simulink model "vipmosaicking"  (R2015b)
settings: Solver=FixedStepDiscrete  StartTime=0.0  StopTime=inf  RelTol=1e-3
undefined symbols (not defined in the file or in its folder): fspecial, gray, imresize, Rec, SDTV
libraries: simulink x5, visiongeotforms x4, visionsinks x2, visiontextngfix x2, visionanalysis x1, visionstatistics x1, vipmisc x1, visionconversions x1, visionsources x1, dspvision x1
settings Model: FPTRunName=Active  Creator=The MathWorks, Inc.  LastModifiedBy=The MathWorks, Inc.
settings DataIOCC: SaveFormat=Array  SaveOutput=off  SignalLogging=off  SaveTime=off
settings OptimizationCC: ExpressionDepthLimit=2147483647  InitFltsAndDblsToZero=on  EfficientMapNaN2IntZero=off
settings DebuggingCC: CheckSSInitialOutputMsg=off  UnderspecifiedInitializationDetection=Classic  MergeDetectMultiDrivingBlocksExec=none  SolverPrmCheckMsg=warning  InheritedTsInSrcMsg=none  ParameterPrecisionLossMsg=none  FcnCallInpInsideContextMsg=UseLocalSettings  StateNameClashWarn=warning
settings HardwareCC: ProdBitPerPointer=32  ProdLargestAtomicFloat=None  ProdIntDivRoundTo=Undefined  ProdEndianess=Unspecified  ProdWordSize=32  ProdHWDeviceType=32-bit Generic  TargetBitPerLong=64  TargetBitPerPointer=64  TargetLongLongMode=on  TargetIntDivRoundTo=Zero  TargetEndianess=LittleEndian  TargetWordSize=64  TargetHWDeviceType=Generic->MATLAB Host Computer  ProdEqTarget=off
settings GRTTargetCC: GeneratePreprocessorConditionals=Disable all  CombineOutputUpdateFcns=off  GRTInterface=on
settings ConfigComp: CovModelRefEnable=Off  CovSFcnEnable=off

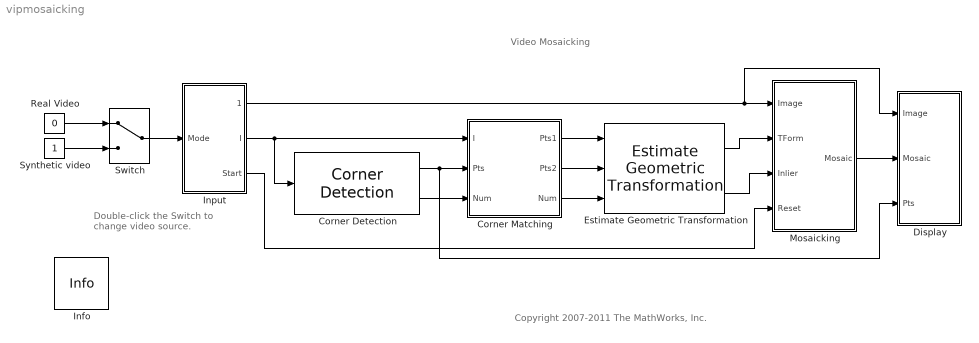
== system vipmosaicking ==
  note: Video Mosaicking
  note: Double-click the Switch to
      | change video source.
  note: Copyright 2007-2011 The MathWorks, Inc.
  Corner Detection : visionanalysis/Corner Detection  method=Local intensity comparison (Rosen & Drummond)  factor=0.04  filter=fspecial('gaussian', [1 5], 1.5)  thrInten=0.1  thrAngle=157.5  output=Obsolete9b  outputInUse=Corner location  maxNum=75  thrMetric=0.001  neighborSize=[21 21]  isOutVarDim=off  accumMode=Binary point scaling  accumWordLength=32  accumFracLength=0  prodOutputMode=Binary point scaling  prodOutputWordLength=32  prodOutputFracLength=0  memoryMode=Binary point scaling  memoryWordLength=32  memoryFracLength=0  firstCoeffMode=Specify word length  firstCoeffWordLength=16  firstCoeffFracLength=16  roundingMode=Floor  overflowMode=off
  Corner Matching : Subsystem  mask(Corner Matching){winLen=9, maxNum=75, threshold=81}
      mask prompts: winLen "Block size used in corner matching:"; maxNum "Maximum number of points:"; threshold "Maximum feature difference for matching points:"
      mask help: Find out matching corners in the current and previous video frames.
  Display : Subsystem
  Estimate Geometric Transformation : visiongeotforms/Estimate Geometric Transformation  tformType=Nonreflective similarity  isRandomSampling=on  algMethod=Random Sample Consensus (RANSAC)  numMethod=Specified value  isStopSampling=off  percentStop=75  distanceAlg=1  distanceGeo=2.5  sampleNum=1000  maxSampleNum=2000  desiredConfidence=99.9  isRefineTForm=off  isOutputInlier=on  outDT4IntInput=Obsolete10a  outDT4IntInputActive=Single  isVarSizeAllowed=off  isReleaseMode=on
  Info : vipmisc/Info  SystemSampleTime=-1
  Input : Subsystem
  Mosaicking : Subsystem  mask(Mosaicking){sizePano=[400 670], originPano=[5 60]}
      mask prompts: sizePano "Size of the mosaic image:"; originPano "Initial image placement (top-left image boundary):"
      mask help: Overlay video frames to create mosaic image.
  Real Video : Constant  Value=0
  Switch : ManualSwitch
  Synthetic video : Constant
  wires:
  Input/1(Image) -> Display/1(Image), Mosaicking/1(Image)
  Input/3(Start) -> Mosaicking/4(Reset)
  Corner Detection/1 -> Display/3(Pts), Corner Matching/2(Pts)
  Corner Detection/2 -> Corner Matching/3(Num)
  Input/2(I) -> Corner Matching/1(I), Corner Detection/1
  Mosaicking/1(Mosaic) -> Display/2(Mosaic)
  Corner Matching/1(Pts1) -> Estimate Geometric Transformation/1
  Corner Matching/2(Pts2) -> Estimate Geometric Transformation/2
  Corner Matching/3("Num ") -> Estimate Geometric Transformation/3
  Estimate Geometric Transformation/2 -> Mosaicking/3(Inlier)
  Estimate Geometric Transformation/1 -> Mosaicking/2(TForm)
  Real Video/1 -> Switch/1
  Synthetic video/1 -> Switch/2
  Switch/1 -> Input/1(Mode)

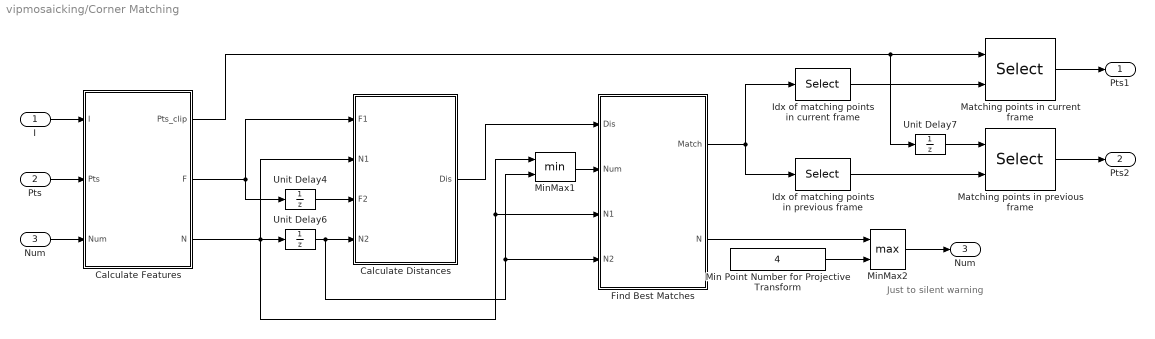
== system vipmosaicking/Corner Matching ==
  note: Just to
      | silent warning
  I : Inport
  Pts : Inport  Port=2
  Num : Inport  Port=3
  Calculate Distances : Subsystem  TreatAsAtomicUnit=on  mask{maxNum=maxNum}
      mask prompts: maxNum "Maximum data number:"
      settings: AttributesFormatString=between features.
  Calculate Features : Subsystem  TreatAsAtomicUnit=on  mask{winLen=winLen, maxNum=maxNum}
      mask prompts: winLen "Neighborhood size:"; maxNum "Maximum number of features:"
  Find Best Matches : Subsystem  TreatAsAtomicUnit=on  mask{maxNum=maxNum, threshold=threshold}
      mask prompts: maxNum "Maximum data number:"
      settings: AttributesFormatString=between the features\nin the current and previous frames
  Idx of matching points in current frame : Selector  NumberOfDimensions=2  IndexMode=Zero-based  InputPortWidth=2  IndexOptions=Select all,Index vector (dialog)  Indices=0,0  OutputSizes=1,1
  Idx of matching points in previous frame : Selector  NumberOfDimensions=2  IndexMode=Zero-based  InputPortWidth=2  IndexOptions=Select all,Index vector (dialog)  Indices=1,1  OutputSizes=1,1
  Matching points in current frame : Selector  NumberOfDimensions=2  IndexMode=Zero-based  InputPortWidth=2  IndexOptions=Index vector (port),Select all  Indices=0,1  OutputSizes=1,1
  Matching points in previous frame : Selector  NumberOfDimensions=2  IndexMode=Zero-based  InputPortWidth=2  IndexOptions=Index vector (port),Select all  Indices=0,1  OutputSizes=1,1
  Min Point Number for Projective Transform : Constant  Value=4  OutDataTypeStr=Inherit: Inherit via back propagation
  MinMax1 : MinMax  Inputs=2
  MinMax2 : MinMax  Function=max  Inputs=2  OutDataTypeStr=Inherit: Inherit via back propagation
  Unit Delay4 : UnitDelay  SampleTime=-1
  Unit Delay6 : UnitDelay  SampleTime=-1
  Unit Delay7 : UnitDelay  SampleTime=-1
  Pts1 : Outport
  Pts2 : Outport  Port=2
  "Num " : Outport  Port=3
  wires:
  Calculate Features/2(F) -> Calculate Distances/1(F1), Unit Delay4/1
  Calculate Features/3(N) -> Calculate Distances/2(N1), Unit Delay6/1, MinMax1/1, Find Best Matches/3(N1)
  Calculate Features/1(Pts_clip) -> Unit Delay7/1, Matching points in current frame/1
  Num/1 -> Calculate Features/3(Num)
  Unit Delay6/1 -> Calculate Distances/4(N2), MinMax1/2, Find Best Matches/4(N2)
  Unit Delay4/1 -> Calculate Distances/3(F2)
  Matching points in previous frame/1 -> Pts2/1
  Matching points in current frame/1 -> Pts1/1
  Unit Delay7/1 -> Matching points in previous frame/1
  Idx of matching points in current frame/1 -> Matching points in current frame/2
  Idx of matching points in previous frame/1 -> Matching points in previous frame/2
  Find Best Matches/1(Match) -> Idx of matching points in previous frame/1, Idx of matching points in current frame/1
  Calculate Distances/1(Dis) -> Find Best Matches/1(Dis)
  I/1 -> Calculate Features/1(I)
  Pts/1 -> Calculate Features/2(Pts)
  Min Point Number for Projective Transform/1 -> MinMax2/2
  Find Best Matches/2(N) -> MinMax2/1
  MinMax2/1 -> "Num "/1
  MinMax1/1 -> Find Best Matches/2(Num)

== system vipmosaicking/Display ==
  Image : Inport
  Mosaic : Inport  Port=2
  Pts : Inport  Port=3
  Corners : visionsinks/Video Viewer  inputType=Obsolete7b  imagePorts=One multidimensional signal  useColorMap=off  colormapValue=gray(256)  specRange=off  minInputVal=0  maxInputVal=255  FigPos=[34 421 347 276]  AxisZoom=on  trueSizedOnce=on  OpenAtMdlStart=on  DefaultConfigurationName=vipscopes.VideoViewerScopeCfg
  Draw Corners : visiontextngfix/Draw Markers  shape=Circle  size=3  fill=off  fillClrSource=Specify via dialog  display=User-specified value  intensity=155  color=[1 0 0]  opacity=1  viewport=Entire image  antialiasing=off  inType=Obsolete  imagePorts=One multidimensional signal  prodOutputMode=Binary point scaling  prodOutputWordLength=32  prodOutputFracLength=14  memoryMode=Specify word length  memoryWordLength=16  memoryFracLength=15  roundingMode=Floor  overflowMode=off
  "Mosaic " : visionsinks/Video Viewer  inputType=Obsolete7b  imagePorts=One multidimensional signal  useColorMap=off  colormapValue=gray(256)  specRange=off  minInputVal=0  maxInputVal=255  FigPos=[316 541 689 427]  AxisZoom=on  trueSizedOnce=on  OpenAtMdlStart=on  DefaultConfigurationName=vipscopes.VideoViewerScopeCfg
  wires:
  Mosaic/1 -> "Mosaic "/1
  Image/1 -> Draw Corners/1
  Draw Corners/1 -> Corners/1
  Pts/1 -> Draw Corners/2

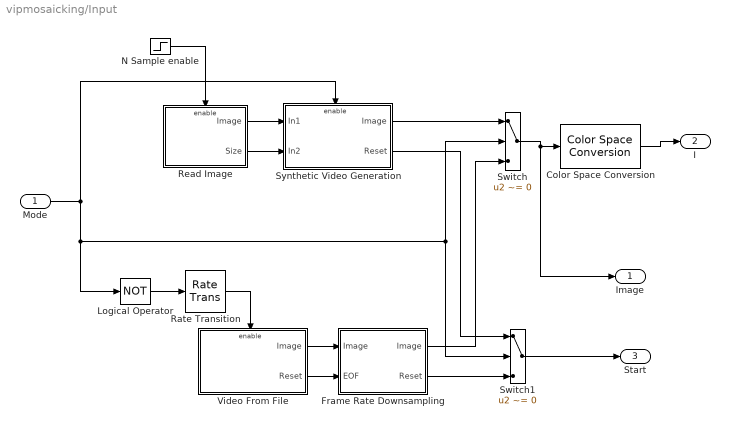
== system vipmosaicking/Input ==
  Mode : Inport
  Color Space Conversion : visionconversions/Color Space  Conversion  conversion=Obsolete  conversionActive=R'G'B' to intensity  wp_str=D65  rec=Rec. 601 (SDTV)  sys=1125/60/2:1  imagePorts=One multidimensional signal
  Frame Rate Downsampling : Subsystem  mask(Select Video Frames){frameRate=5}
      mask prompts: frameRate "N:"
      mask help: Downsample the video sequence by processing every Nth frame.
      mask init:
      | switch frameRate
      |     case 1,
      |         icon = sprintf('Select\nAll Frames');
      |     case 2,
      |         icon = sprintf('Select Every\n2nd Frame');
      |     case 3,
      |         icon = sprintf('Select Every\n3rd Frame');
      |     otherwise,
      |         icon = sprintf('Select Every\n%dth Frame',frameRate);
      | end
      mask Display: disp(icon);
  Logical Operator : Logic  Operator=NOT  AllPortsSameDT=off  OutDataTypeStr=boolean
  N Sample enable : Step  Time=eps  Before=1  After=0
  Rate Transition : RateTransition  OutPortSampleTimeOpt=Inherit
  Read Image : Subsystem
      settings: AttributesFormatString=Load image only at the beginning of simulation
  Switch : Switch  Criteria=u2 ~= 0
  Switch1 : Switch  Criteria=u2 ~= 0
  Synthetic Video Generation : Subsystem  mask(Synthetic Video Generation){dimen=[240 320], origin=[765 509], velocity=[10 5], varVelocity=[5 2], varCorner=[10 10], rotation=1, varRotation=0.2}
      mask prompts: dimen "Size of the synthetic image:"; origin "Initial image center:"; varVelocity "Variance of velocity:"; varCorner "Variance of corner location:"; rotation "Rotation speed (in degrees):"; varRotation "Variation of rotation (in degrees):"
      mask help: Generates a synthetic video.
  Video From File : Subsystem
  Image : Outport
  I : Outport  Port=2
  Start : Outport  Port=3
  wires:
  Color Space Conversion/1 -> I/1
  Switch1/1 -> Start/1
  Switch/1 -> Image/1, Color Space Conversion/1
  Logical Operator/1 -> Rate Transition/1
  Rate Transition/1 -> Video From File/Enable
  Synthetic Video Generation/2(Reset) -> Switch1/1
  Synthetic Video Generation/1(Image) -> Switch/1
  Mode/1 -> Logical Operator/1, Switch/2, Switch1/2, Synthetic Video Generation/Enable
  Video From File/1(Image) -> Frame Rate Downsampling/1(Image)
  Video From File/2(Reset) -> Frame Rate Downsampling/2(EOF)
  Frame Rate Downsampling/1("Image ") -> Switch/3
  Frame Rate Downsampling/2(Reset) -> Switch1/3
  Read Image/2(Size) -> Synthetic Video Generation/2(In2)
  N Sample enable/1 -> Read Image/Enable
  Read Image/1(Image) -> Synthetic Video Generation/1(In1)

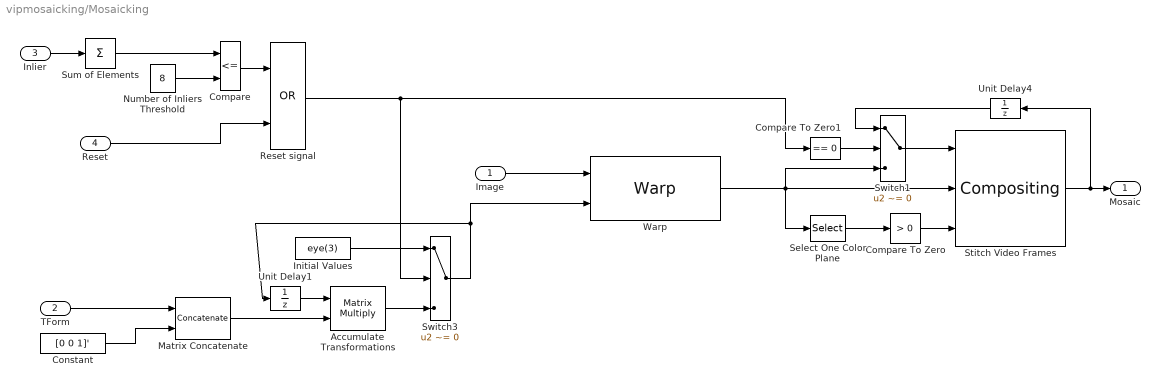
== system vipmosaicking/Mosaicking ==
  Image : Inport
  TForm : Inport  Port=2
  Inlier : Inport  Port=3
  Reset : Inport  Port=4
  Accumulate Transformations : Product  Multiplication=Matrix(*)  RndMeth=Zero  InputSameDT=on
  Compare : RelationalOperator  Operator=<=  OutDataTypeStr=boolean  ZeroCross=off  InputSameDT=on
  Compare To Zero : simulink/Logic and Bit Operations/Compare To Zero  relop=>  OutDataTypeStr=boolean  ZeroCross=off
  Compare To Zero1 : simulink/Logic and Bit Operations/Compare To Zero  relop===  OutDataTypeStr=boolean  ZeroCross=off
  Constant : Constant  Value=[0 0 1]'  VectorParams1D=off  OutDataTypeStr=Inherit: Inherit via back propagation
  Initial Values : Constant  Value=eye(3)  OutDataTypeStr=Inherit: Inherit via back propagation  SampleTime=-1
  Matrix Concatenate : Concatenate  Mode=Multidimensional array  ConcatenateDimension=2
  Number of Inliers Threshold : Constant  Value=8  OutDataTypeStr=Inherit: Inherit via back propagation  SampleTime=-1
  Reset signal : Logic  Operator=OR  AllPortsSameDT=off  OutDataTypeStr=boolean
      settings: AttributesFormatString=Restart mosaicking when the video started\nor when no enough inliers were found.
  Select One Color Plane : Selector  NumberOfDimensions=3  InputPortWidth=3  IndexOptions=Select all,Select all,Index vector (dialog)  Indices=40,10,1  OutputSizes=240,320,1
  Stitch Video Frames : visiontextngfix/Compositing  operation=Binary mask  bFacSrc=Specify via dialog  mFacSrc=Input port  bFactor=0.2  mFactor=1  source=Specify via dialog  coordinates=[0 0]  prodOutputMode=Binary point scaling  prodOutputWordLength=32  prodOutputFracLength=10  roundingMode=Floor  overflowMode=off
  Sum of Elements : Sum  Inputs=+
  Switch1 : Switch  Criteria=u2 ~= 0  ZeroCross=off  InputSameDT=on
  Switch3 : Switch  Criteria=u2 ~= 0  ZeroCross=off  InputSameDT=on
  Unit Delay1 : UnitDelay  SampleTime=-1
  Unit Delay4 : UnitDelay  SampleTime=-1
  Warp : visiongeotforms/Warp  TransformMatrixSource=Input port  TransformMatrix=eye( 3 )  InterpolationMethod=Bilinear  BackgroundFillValue=0  OutputImagePositionSource=Custom  OutputImagePosition=[-originPano, sizePano([2,1])]  ROIInputPort=off  ROIValidityOutputPort=off  SimulateUsing=Interpreted execution
  Mosaic : Outport
  wires:
  Reset/1 -> Reset signal/2
  Compare/1 -> Reset signal/1
  Unit Delay4/1 -> Switch1/1
  Inlier/1 -> Sum of Elements/1
  Number of Inliers Threshold/1 -> Compare/2
  Sum of Elements/1 -> Compare/1
  Switch3/1 -> Warp/2, Unit Delay1/1
  Reset signal/1 -> Switch3/2, Compare To Zero1/1
  Accumulate Transformations/1 -> Switch3/3
  Unit Delay1/1 -> Accumulate Transformations/1
  Initial Values/1 -> Switch3/1
  Select One Color Plane/1 -> Compare To Zero/1
  Warp/1 -> Switch1/3, Select One Color Plane/1, Stitch Video Frames/2
  Stitch Video Frames/1 -> Unit Delay4/1, Mosaic/1
  Switch1/1 -> Stitch Video Frames/1
  Compare To Zero/1 -> Stitch Video Frames/3
  Compare To Zero1/1 -> Switch1/2
  Image/1 -> Warp/1
  TForm/1 -> Matrix Concatenate/1
  Constant/1 -> Matrix Concatenate/2
  Matrix Concatenate/1 -> Accumulate Transformations/2

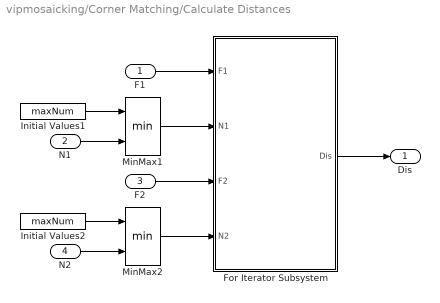
== system vipmosaicking/Corner Matching/Calculate Distances ==
  F1 : Inport
  N1 : Inport  Port=2
  F2 : Inport  Port=3
  N2 : Inport  Port=4
  For Iterator Subsystem : Subsystem  TreatAsAtomicUnit=on
  Initial Values1 : Constant  Value=maxNum  OutDataTypeStr=Inherit: Inherit via back propagation  SampleTime=-1
  Initial Values2 : Constant  Value=maxNum  OutDataTypeStr=Inherit: Inherit via back propagation  SampleTime=-1
  MinMax1 : MinMax  Inputs=2
  MinMax2 : MinMax  Inputs=2
  Dis : Outport
  wires:
  MinMax2/1 -> For Iterator Subsystem/4(N2)
  F2/1 -> For Iterator Subsystem/3(F2)
  MinMax1/1 -> For Iterator Subsystem/2(N1)
  F1/1 -> For Iterator Subsystem/1(F1)
  For Iterator Subsystem/1(Dis) -> Dis/1
  N2/1 -> MinMax2/2
  Initial Values2/1 -> MinMax2/1
  N1/1 -> MinMax1/2
  Initial Values1/1 -> MinMax1/1

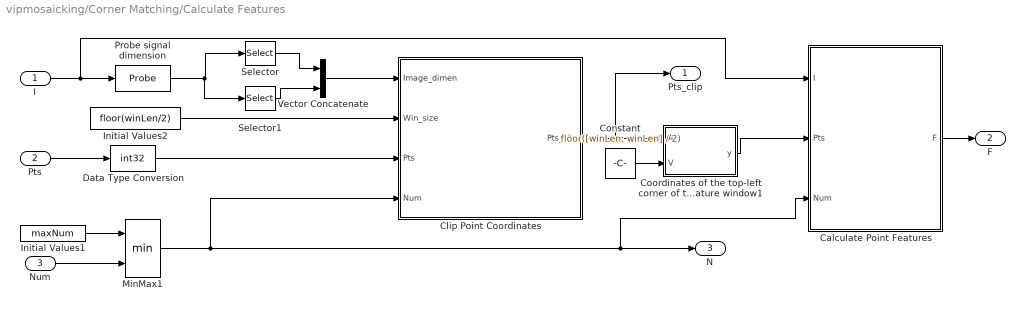
== system vipmosaicking/Corner Matching/Calculate Features ==
  I : Inport
  Pts : Inport  Port=2
  Num : Inport  Port=3
  Calculate Point Features : Subsystem
  Clip Point Coordinates : Subsystem
  Constant : Constant  Value=floor([winLen; winLen] / 2)  OutDataTypeStr=int32
  Coordinates of the top-left corner of the feature window1 : MATLAB Function  TreatAsAtomicUnit=on
  Data Type Conversion : DataTypeConversion  OutDataTypeStr=int32
  Initial Values1 : Constant  Value=maxNum  OutDataTypeStr=Inherit: Inherit via back propagation  SampleTime=-1
  Initial Values2 : Constant  Value=floor(winLen/2)  OutDataTypeStr=Inherit: Inherit via back propagation  SampleTime=-1
  MinMax1 : MinMax  Inputs=2
  Probe signal dimension : Probe  ProbeWidth=off  ProbeSampleTime=off  ProbeComplexSignal=off  ProbeSignalDimensions=on  ProbeDimensionsDataType=int32
  Selector : Selector  InputPortWidth=2  IndexOptions=Index vector (dialog)  Indices=2  OutputSizes=1
  Selector1 : Selector  InputPortWidth=2  IndexOptions=Index vector (dialog)  Indices=1  OutputSizes=1
  Vector Concatenate : Concatenate
  Pts_clip : Outport
  F : Outport  Port=2
  N : Outport  Port=3
  wires:
  Data Type Conversion/1 -> Clip Point Coordinates/3(Pts)
  MinMax1/1 -> N/1, Calculate Point Features/3(Num), Clip Point Coordinates/4(Num)
  Coordinates of the top-left corner of the feature window1/1(y) -> Calculate Point Features/2(Pts)
  Clip Point Coordinates/1(Pts_clip) -> Pts_clip/1, Coordinates of the top-left corner of the feature window1/1(A)
  Pts/1 -> Data Type Conversion/1
  Initial Values2/1 -> Clip Point Coordinates/2(Win_size)
  I/1 -> Calculate Point Features/1(I), Probe signal dimension/1
  Initial Values1/1 -> MinMax1/1
  Num/1 -> MinMax1/2
  Calculate Point Features/1(F) -> F/1
  Probe signal dimension/1 -> Selector1/1, Selector/1
  Selector/1 -> Vector Concatenate/1
  Vector Concatenate/1 -> Clip Point Coordinates/1(Image_dimen)
  Selector1/1 -> Vector Concatenate/2
  Constant/1 -> Coordinates of the top-left corner of the feature window1/2(V)

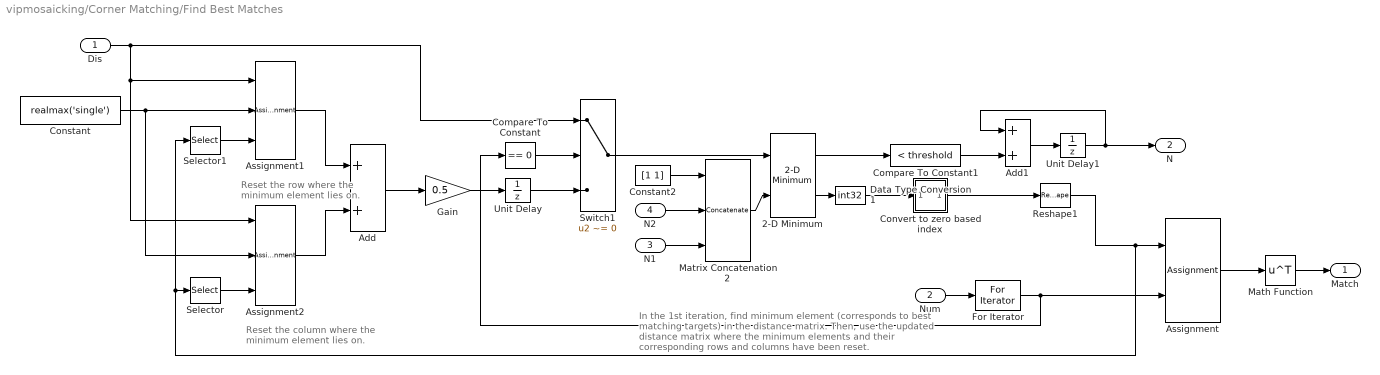
== system vipmosaicking/Corner Matching/Find Best Matches ==
  note: In the 1st iteration, find minimum element (corresponds to
      | best matching targets) in the distance matrix. Then, use the
      | updated distance matrix where the minimum elements and
      | their  corresponding rows and columns have been reset.
  note: Reset the column where the
      | minimum element lies on.
  note: Reset the row where the
      | minimum element lies on.
  Dis : Inport
  Num : Inport  Port=2
  N1 : Inport  Port=3
  N2 : Inport  Port=4
  2-D Minimum : visionstatistics/2-D Minimum  fcn=Value and Index  reset=None  indexBase=One  operateOver=Entire input  Dimension=1  colComp=on  operation=minimum  roiEnable=on  roiType=Rectangles  roiPortion=Entire ROI  roiOutput=Individual statistics for each ROI  roiFlag=off  accumDataTypeStr=Inherit: Same as product output  accumLastDataTypeStr=Inherit: Same as product output  roundingMode=Floor  overflowMode=off
  Add : Sum
  Add1 : Sum  OutDataTypeStr=int32
  Assignment : Assignment  NumberOfDimensions=2  IndexMode=Zero-based  OutputInitialize=Specify size for each dimension in table  IndexOptions=Assign all,Index vector (port)  Indices=-1,-1  OutputSizes=2,maxNum
  Assignment1 : Assignment  NumberOfDimensions=2  IndexMode=Zero-based  IndexOptions=Index vector (port),Assign all  Indices=1,-1  OutputSizes=1,1
  Assignment2 : Assignment  NumberOfDimensions=2  IndexMode=Zero-based  IndexOptions=Assign all,Index vector (port)  Indices=-1,-1  OutputSizes=1,1
  Compare To Constant : simulink/Logic and Bit Operations/Compare To Constant  relop===  const=0  OutDataTypeStr=boolean  ZeroCross=off
  Compare To Constant1 : simulink/Logic and Bit Operations/Compare To Constant  relop=<  const=threshold  OutDataTypeStr=uint8  ZeroCross=off
  Constant : Constant  Value=realmax('single')  VectorParams1D=off  OutDataTypeStr=Inherit: Inherit via back propagation
  Constant2 : Constant  Value=[1 1]  VectorParams1D=off  OutDataTypeStr=Inherit: Inherit via back propagation
  "Convert to zero based index " : Subsystem
  Data Type Conversion1 : DataTypeConversion  OutDataTypeStr=int32  SaturateOnIntegerOverflow=on  RndMeth=Zero
  For Iterator : ForIterator  ResetStates=reset  IterationSource=external  IterationLimit=expLaneNum  IndexMode=Zero-based
  Gain : Gain  Gain=0.5
  Math Function : Math  Operator=transpose  SaturateOnIntegerOverflow=on
  Matrix Concatenation2 : Concatenate  NumInputs=3  Mode=Multidimensional array  ConcatenateDimension=2
  Reshape1 : Reshape  OutputDimensionality=Column vector (2-D)
  Selector : Selector  IndexMode=Zero-based  InputPortWidth=2  IndexOptions=Index vector (dialog)  Indices=1  OutputSizes=1
  Selector1 : Selector  IndexMode=Zero-based  InputPortWidth=2  IndexOptions=Index vector (dialog)  Indices=0  OutputSizes=1
  Switch1 : Switch  Criteria=u2 ~= 0
  Unit Delay : UnitDelay  SampleTime=-1
  Unit Delay1 : UnitDelay  SampleTime=-1
  Match : Outport
  N : Outport  Port=2
  wires:
  Gain/1 -> Unit Delay/1
  Compare To Constant1/1 -> Add1/2
  Unit Delay1/1 -> Add1/1, N/1
  Add1/1 -> Unit Delay1/1
  Num/1 -> For Iterator/1
  Compare To Constant/1 -> Switch1/2
  For Iterator/1 -> Compare To Constant/1, Assignment/2
  Switch1/1 -> 2-D Minimum/1
  Dis/1 -> Switch1/1, Assignment2/1, Assignment1/1
  Unit Delay/1 -> Switch1/3
  Assignment/1 -> Math Function/1
  Selector1/1 -> Assignment1/3
  Assignment1/1 -> Add/1
  Assignment2/1 -> Add/2
  Add/1 -> Gain/1
  Constant/1 -> Assignment1/2, Assignment2/2
  Selector/1 -> Assignment2/3
  Math Function/1 -> Match/1
  Matrix Concatenation2/1 -> 2-D Minimum/2
  Constant2/1 -> Matrix Concatenation2/1
  2-D Minimum/2 -> Data Type Conversion1/1
  2-D Minimum/1 -> Compare To Constant1/1
  N2/1 -> Matrix Concatenation2/2
  N1/1 -> Matrix Concatenation2/3
  Data Type Conversion1/1 -> "Convert to zero based index "/1(In1)
  "Convert to zero based index "/1(Out1) -> Reshape1/1
  Reshape1/1 -> Assignment/1, Selector/1, Selector1/1

== system vipmosaicking/Input/Frame Rate Downsampling ==
  Image : Inport
  EOF : Inport  Port=2
  Compare To Zero : simulink/Logic and Bit Operations/Compare To Zero  relop=>  OutDataTypeStr=boolean  ZeroCross=off
  Data Type Conversion : DataTypeConversion  OutDataTypeStr=single
  Discrete FIR Filter : DiscreteFir  Coefficients=ones(1, frameRate)
  Downsample : DownSample  N=frameRate  RateOptions=Allow multirate processing
  Downsample3 : DownSample  N=frameRate  RateOptions=Allow multirate processing
  Unit Delay : UnitDelay  InitialCondition=1  SampleTime=-1
  "Image " : Outport
  Reset : Outport  Port=2
  wires:
  Discrete FIR Filter/1 -> Compare To Zero/1
  Data Type Conversion/1 -> Discrete FIR Filter/1
  Compare To Zero/1 -> Unit Delay/1
  Downsample3/1 -> Reset/1
  EOF/1 -> Data Type Conversion/1
  Unit Delay/1 -> Downsample3/1
  Image/1 -> Downsample/1
  Downsample/1 -> "Image "/1

== system vipmosaicking/Input/Read Image ==
  Enable : EnablePort  PropagateVarSize=During execution
  Image From Workspace : visionsources/Image From Workspace  Tag=vipblks_nd  ImageValue=imresize(imread('concordaerial.png'), 0.5)  Ts=inf  imagePorts=One multidimensional signal  ImageDataType=single  Signed=on  WordLength=16  sdImageDataType=sfix(16)  FractionLengthMode=User-defined  FractionLength=15  OutPortLabels=R|G|B
  Probe : Probe  ProbeWidth=off  ProbeSampleTime=off  ProbeComplexSignal=off  ProbeSignalDimensions=on  ProbeDimensionsDataType=single
  Image : Outport  InitialOutput=0
  Size : Outport  Port=2
  wires:
  Image From Workspace/1 -> Probe/1, Image/1
  Probe/1 -> Size/1

== system vipmosaicking/Input/Synthetic Video Generation ==
  In1 : Inport
  In2 : Inport  Port=2
  Enable : EnablePort  PropagateVarSize=During execution
  Synthesize Video : Subsystem  mask{dimen=dimen, origin=origin, velocity=velocity, varVelocity=varVelocity, varCorner=varCorner, rotation=rotation, varRotation=varRotation}
      mask prompts: dimen "Size of the synthetic image:"; origin "Initial image center:"; varVelocity "Variance of velocity:"; varCorner "Variance of corner location:"; rotation "Rotation speed:"; varRotation "Variation of rotation:"
  Image : Outport
  Reset : Outport  Port=2  InitialOutput=1
  wires:
  Synthesize Video/2(Reset) -> Reset/1
  Synthesize Video/1(Image) -> Image/1
  In2/1 -> Synthesize Video/2(Size)
  In1/1 -> Synthesize Video/1("Image ")

== system vipmosaicking/Input/Video From File ==
  Enable : EnablePort  PropagateVarSize=During execution
  From Multimedia File : dspvision/From Multimedia File  inputFilename=vipmosaicking.avi  loop=on  numPlays=inf  outputStreams=Video only  videoDataType=single  audioDataType=int16  inheritSampleTime=on  userDefinedSampleTime=1/30  noAudioOutput=off  isIntensityVideo=off  fourcc=RGB  colorVideoFormat=One multidimensional signal  outputEOF=on  dataOrg=Column-major  audioFrameSize=1024  computeAudioFrameSize=off  outSamplingMode=Frame based
  Image : Outport
  Reset : Outport  Port=2
  wires:
  From Multimedia File/1 -> Image/1
  From Multimedia File/2 -> Reset/1

== system vipmosaicking/Corner Matching/Calculate Distances/For Iterator Subsystem ==
  F1 : Inport
  N1 : Inport  Port=2
  F2 : Inport  Port=3
  N2 : Inport  Port=4
  For Iterator : ForIterator  IterationSource=external  IndexMode=Zero-based
  For Iterator Subsystem : Subsystem  TreatAsAtomicUnit=on
  Select feature for 1 corner : Selector  NumberOfDimensions=2  IndexMode=Zero-based  InputPortWidth=2  IndexOptions=Index vector (port),Select all  Indices=0,1  OutputSizes=1,1
  Update feature for a corner : Assignment  NumberOfDimensions=2  IndexMode=Zero-based  OutputInitialize=Specify size for each dimension in table  IndexOptions=Assign all,Index vector (port)  Indices=1,1  OutputSizes=maxNum,maxNum
  Dis : Outport
  wires:
  Update feature for a corner/1 -> Dis/1
  N1/1 -> For Iterator Subsystem/2(N1)
  F1/1 -> For Iterator Subsystem/1(F1)
  Select feature for 1 corner/1 -> For Iterator Subsystem/3(f2)
  F2/1 -> Select feature for 1 corner/1
  For Iterator/1 -> Select feature for 1 corner/2, Update feature for a corner/2
  N2/1 -> For Iterator/1
  For Iterator Subsystem/1(Dis) -> Update feature for a corner/1

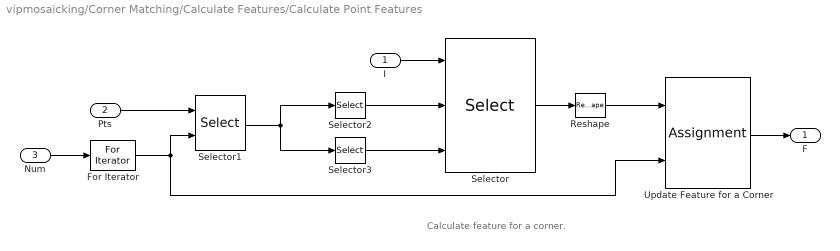
== system vipmosaicking/Corner Matching/Calculate Features/Calculate Point Features ==
  note: Calculate feature for a corner.
  I : Inport
  Pts : Inport  Port=2
  Num : Inport  Port=3
  For Iterator : ForIterator  IterationSource=external  IndexMode=Zero-based
  Reshape : Reshape  OutputDimensionality=Row vector (2-D)
  Selector : Selector  NumberOfDimensions=2  IndexMode=Zero-based  InputPortWidth=3  IndexOptions=Starting index (port),Starting index (port)  Indices=[1 3],1  OutputSizes=winLen,winLen
  Selector1 : Selector  NumberOfDimensions=2  IndexMode=Zero-based  InputPortWidth=3  IndexOptions=Index vector (port),Select all  Indices=[1 3],1  OutputSizes=9,9
  Selector2 : Selector  IndexMode=Zero-based  InputPortWidth=2  IndexOptions=Index vector (dialog)  Indices=1  OutputSizes=9
  Selector3 : Selector  IndexMode=Zero-based  InputPortWidth=2  IndexOptions=Index vector (dialog)  Indices=0  OutputSizes=9
  Update Feature for a Corner : Assignment  NumberOfDimensions=2  IndexMode=Zero-based  OutputInitialize=Specify size for each dimension in table  IndexOptions=Index vector (port),Assign all  Indices=1,1  OutputSizes=maxNum,winLen^2
  F : Outport
  wires:
  Selector3/1 -> Selector/3
  Selector2/1 -> Selector/2
  Num/1 -> For Iterator/1
  Update Feature for a Corner/1 -> F/1
  Pts/1 -> Selector1/1
  I/1 -> Selector/1
  Reshape/1 -> Update Feature for a Corner/1
  Selector/1 -> Reshape/1
  Selector1/1 -> Selector2/1, Selector3/1
  For Iterator/1 -> Update Feature for a Corner/2, Selector1/2

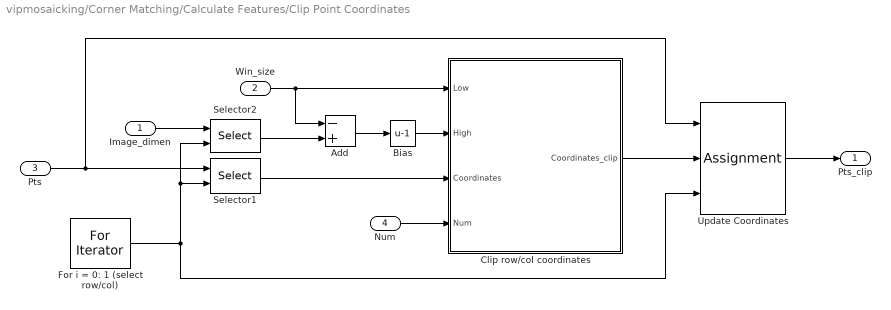
== system vipmosaicking/Corner Matching/Calculate Features/Clip Point Coordinates ==
  Image_dimen : Inport
  Win_size : Inport  Port=2
  Pts : Inport  Port=3
  Num : Inport  Port=4
  Add : Sum  Inputs=-+
  Bias : Bias  Bias=-1
  Clip row/col coordinates : Subsystem
  For i = 0: 1 (select row/col) : ForIterator  IterationLimit=2  IndexMode=Zero-based
  Selector1 : Selector  NumberOfDimensions=2  IndexMode=Zero-based  InputPortWidth=3  IndexOptions=Select all,Index vector (port)  Indices=[1 3],1  OutputSizes=9,9
  Selector2 : Selector  IndexMode=Zero-based  InputPortWidth=2  IndexOptions=Index vector (port)  Indices=[1 3]  OutputSizes=9
  Update Coordinates : Assignment  NumberOfDimensions=2  IndexMode=Zero-based  IndexOptions=Assign all,Index vector (port)  Indices=1,1  OutputSizes=81,50
  Pts_clip : Outport
  wires:
  Selector2/1 -> Add/2
  For i = 0: 1 (select row/col)/1 -> Selector1/2, Selector2/2, Update Coordinates/3
  Clip row/col coordinates/1(Coordinates_clip) -> Update Coordinates/2
  Bias/1 -> Clip row/col coordinates/2(High)
  Update Coordinates/1 -> Pts_clip/1
  Num/1 -> Clip row/col coordinates/4(Num)
  Selector1/1 -> Clip row/col coordinates/3(Coordinates)
  Win_size/1 -> Add/1, Clip row/col coordinates/1(Low)
  Add/1 -> Bias/1
  Image_dimen/1 -> Selector2/1
  Pts/1 -> Update Coordinates/1, Selector1/1

== system vipmosaicking/Corner Matching/Find Best Matches/Convert to zero based index  ==
  In1 : Inport
  Constant : Constant
  Selector : Selector  NumberOfDimensions=2  InputPortWidth=3  IndexOptions=Select all,Index vector (dialog)  Indices=[1 3],[2 1]  OutputSizes=1,1
  Subtract : Sum  Inputs=+-
  Out1 : Outport
  wires:
  Selector/1 -> Subtract/1
  Constant/1 -> Subtract/2
  In1/1 -> Selector/1
  Subtract/1 -> Out1/1

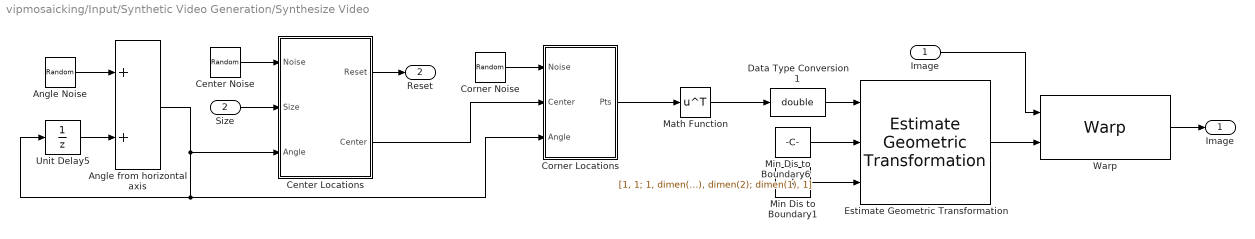
== system vipmosaicking/Input/Synthetic Video Generation/Synthesize Video ==
  "Image " : Inport
  Size : Inport  Port=2
  Angle Noise : RandomNumber  Mean=rotation * pi / 180  Variance=varRotation * pi / 180  Seed=rotation
  Angle from horizontal axis : Sum
  Center Locations : Subsystem
  Center Noise : RandomNumber  Mean=[1 1]  Variance=[1; 1]  Seed=velocity
  Corner Locations : Subsystem
  Corner Noise : RandomNumber  Mean=zeros(2, 4)  Variance=[ones(1,4) * varCorner(1); ones(1,4) * varCorner(2)]
  Data Type Conversion1 : DataTypeConversion  OutDataTypeStr=double
  Estimate Geometric Transformation : visiongeotforms/Estimate Geometric Transformation  tformType=Projective  isRandomSampling=off  algMethod=Random Sample Consensus (RANSAC)  numMethod=Specified value  isStopSampling=off  percentStop=75  distanceAlg=1.5  distanceGeo=1.5  sampleNum=100  maxSampleNum=200  desiredConfidence=99  isRefineTForm=off  isOutputInlier=off  outDT4IntInput=Obsolete10a  outDT4IntInputActive=Single  isVarSizeAllowed=off  isReleaseMode=on
  Math Function : Math  Operator=transpose  SaturateOnIntegerOverflow=on
  Min Dis to Boundary1 : Constant  Value=4  OutDataTypeStr=Inherit: Inherit via back propagation
  Min Dis to Boundary6 : Constant  Value=[1, 1; 1, dimen(2); dimen(1), dimen(2); dimen(1), 1]  OutDataTypeStr=double
  Unit Delay5 : UnitDelay  InitialCondition=-pi/12  SampleTime=-1
  Warp : visiongeotforms/Warp  TransformMatrixSource=Input port  TransformMatrix=eye( 3 )  InterpolationMethod=Bilinear  BackgroundFillValue=0  OutputImagePositionSource=Custom  OutputImagePosition=[ 1, 1, dimen([2,1])]  ROIInputPort=off  ROIValidityOutputPort=off  SimulateUsing=Interpreted execution
  Image : Outport
  Reset : Outport  Port=2
  wires:
  Center Noise/1 -> Center Locations/1(Noise)
  Corner Noise/1 -> Corner Locations/1(Noise)
  Angle from horizontal axis/1 -> Center Locations/3(Angle), Corner Locations/3(Angle), Unit Delay5/1
  Angle Noise/1 -> Angle from horizontal axis/1
  Center Locations/1(Reset) -> Reset/1
  Unit Delay5/1 -> Angle from horizontal axis/2
  Size/1 -> Center Locations/2(Size)
  Center Locations/2(Center) -> Corner Locations/2(Center)
  "Image "/1 -> Warp/1
  Min Dis to Boundary6/1 -> Estimate Geometric Transformation/2
  Min Dis to Boundary1/1 -> Estimate Geometric Transformation/3
  Warp/1 -> Image/1
  Data Type Conversion1/1 -> Estimate Geometric Transformation/1
  Estimate Geometric Transformation/1 -> Warp/2
  Corner Locations/1(Pts) -> Math Function/1
  Math Function/1 -> Data Type Conversion1/1

== system vipmosaicking/Corner Matching/Calculate Distances/For Iterator Subsystem/For Iterator Subsystem ==
  F1 : Inport
  N1 : Inport  Port=2
  f2 : Inport  Port=3
  Distance between two feature vectors : Subsystem
  For Iterator : ForIterator  IterationSource=external  IndexMode=Zero-based
  Select feature for 1 corner : Selector  NumberOfDimensions=2  IndexMode=Zero-based  InputPortWidth=2  IndexOptions=Index vector (port),Select all  Indices=0,1  OutputSizes=1,1
  Update feature for a corner : Assignment  NumberOfDimensions=2  IndexMode=Zero-based  OutputInitialize=Specify size for each dimension in table  IndexOptions=Index vector (port),Assign all  Indices=1,1  OutputSizes=maxNum,1
  Dis : Outport
  wires:
  Select feature for 1 corner/1 -> Distance between two feature vectors/1(f1)
  f2/1 -> Distance between two feature vectors/2(f2)
  Update feature for a corner/1 -> Dis/1
  F1/1 -> Select feature for 1 corner/1
  For Iterator/1 -> Select feature for 1 corner/2, Update feature for a corner/2
  N1/1 -> For Iterator/1
  Distance between two feature vectors/1(dis) -> Update feature for a corner/1

== system vipmosaicking/Corner Matching/Calculate Features/Clip Point Coordinates/Clip row//col coordinates ==
  Low : Inport
  High : Inport  Port=2
  Coordinates : Inport  Port=3
  Num : Inport  Port=4
  Clip a Coordinate : Subsystem
  For Iterator : ForIterator  IterationSource=external  IterationLimit=2  IndexMode=Zero-based
  Select Coordinate of a Point : Selector  NumberOfDimensions=2  IndexMode=Zero-based  InputPortWidth=3  IndexOptions=Index vector (port),Select all  Indices=[1 3],1  OutputSizes=9,1
  Update Feature for a Corner : Assignment  NumberOfDimensions=2  IndexMode=Zero-based  IndexOptions=Index vector (port),Assign all  Indices=1,1  OutputSizes=81,50
  Coordinates_clip : Outport
  wires:
  Clip a Coordinate/1(Coordinate_clip) -> Update Feature for a Corner/2
  Update Feature for a Corner/1 -> Coordinates_clip/1
  High/1 -> Clip a Coordinate/2(High)
  Low/1 -> Clip a Coordinate/1(Low)
  Select Coordinate of a Point/1 -> Clip a Coordinate/3(Coordinate)
  Num/1 -> For Iterator/1
  Coordinates/1 -> Update Feature for a Corner/1, Select Coordinate of a Point/1
  For Iterator/1 -> Select Coordinate of a Point/2, Update Feature for a Corner/3

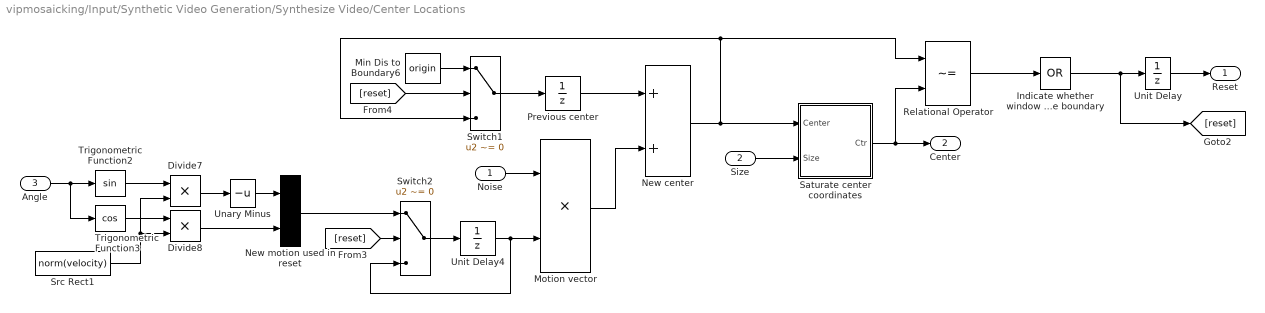
== system vipmosaicking/Input/Synthetic Video Generation/Synthesize Video/Center Locations ==
  Noise : Inport
  Size : Inport  Port=2
  Angle : Inport  Port=3
  Divide7 : Product  Inputs=**
  Divide8 : Product  Inputs=**
  Indicate whether window hit image boundary : Logic  Operator=OR  Inputs=1  AllPortsSameDT=off  OutDataTypeStr=boolean
  Min Dis to Boundary6 : Constant  Value=origin
  Motion vector : Product  Inputs=**
  New center : Sum
  New motion used in reset : Concatenate
  Previous center : UnitDelay  InitialCondition=origin  SampleTime=-1
  Relational Operator : RelationalOperator  Operator=~=  OutDataTypeStr=boolean
  Saturate center coordinates : Subsystem
  Src Rect1 : Constant  Value=norm(velocity)  VectorParams1D=off  OutDataTypeStr=Inherit: Inherit via back propagation
  Switch1 : Switch  Criteria=u2 ~= 0
  Switch2 : Switch  Criteria=u2 ~= 0
  Trigonometric Function2 : Trigonometry
  Trigonometric Function3 : Trigonometry  Operator=cos
  Unary Minus : UnaryMinus
  Unit Delay : UnitDelay  InitialCondition=1  SampleTime=-1
  Unit Delay4 : UnitDelay  InitialCondition=velocity  SampleTime=-1
  Reset : Outport
  Center : Outport  Port=2
  wires:
  Noise/1 -> Motion vector/1
  Motion vector/1 -> New center/2
  Unit Delay4/1 -> Motion vector/2, Switch2/3
  Previous center/1 -> New center/1
  [reset] -> Switch1/2
  [reset] -> Switch2/2
  Divide7/1 -> Unary Minus/1
  Unary Minus/1 -> New motion used in reset/1
  Divide8/1 -> New motion used in reset/2
  Src Rect1/1 -> Divide8/2, Divide7/2
  Switch1/1 -> Previous center/1
  Min Dis to Boundary6/1 -> Switch1/1
  Switch2/1 -> Unit Delay4/1
  New motion used in reset/1 -> Switch2/1
  Trigonometric Function3/1 -> Divide8/1
  Trigonometric Function2/1 -> Divide7/1
  Angle/1 -> Trigonometric Function3/1, Trigonometric Function2/1
  Relational Operator/1 -> Indicate whether window hit image boundary/1
  Indicate whether window hit image boundary/1 -> [reset], Unit Delay/1
  Saturate center coordinates/1(Ctr) -> Center/1, Relational Operator/2
  Size/1 -> Saturate center coordinates/2(Size)
  New center/1 -> Saturate center coordinates/1(Center), Switch1/3, Relational Operator/1
  Unit Delay/1 -> Reset/1

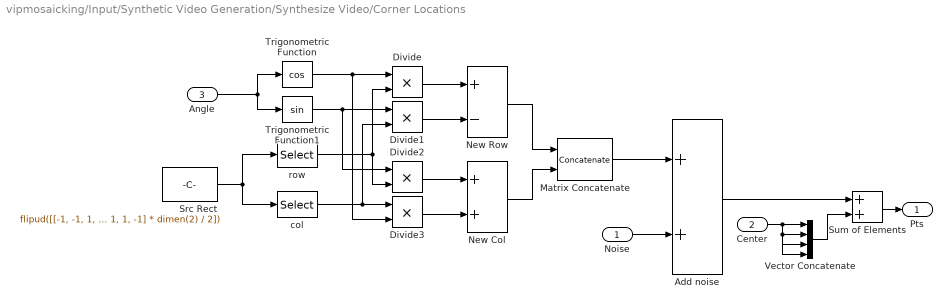
== system vipmosaicking/Input/Synthetic Video Generation/Synthesize Video/Corner Locations ==
  Noise : Inport
  Center : Inport  Port=2
  Angle : Inport  Port=3
  Add noise : Sum
  Divide{,1..3} (4 alike) : Product  Inputs=**
  Matrix Concatenate : Concatenate  Mode=Multidimensional array
  New Col : Sum
  New Row : Sum  Inputs=+-
  Src Rect : Constant  Value=flipud([[-1, -1, 1, 1] * dimen(1) / 2; [-1, 1, 1, -1] * dimen(2) / 2])
  Sum of Elements : Sum
  Trigonometric Function : Trigonometry  Operator=cos
  Trigonometric Function1 : Trigonometry
  Vector Concatenate : Concatenate  NumInputs=4  Mode=Multidimensional array  ConcatenateDimension=2
  col : Selector  NumberOfDimensions=2  IndexMode=Zero-based  InputPortWidth=3  IndexOptions=Index vector (dialog),Select all  Indices=1,1  OutputSizes=1,1
  row : Selector  NumberOfDimensions=2  IndexMode=Zero-based  InputPortWidth=3  IndexOptions=Index vector (dialog),Select all  Indices=0,1  OutputSizes=1,1
  Pts : Outport
  wires:
  Noise/1 -> Add noise/2
  Sum of Elements/1 -> Pts/1
  Src Rect/1 -> col/1, row/1
  Divide2/1 -> New Col/1
  Divide3/1 -> New Col/2
  New Row/1 -> Matrix Concatenate/1
  New Col/1 -> Matrix Concatenate/2
  Matrix Concatenate/1 -> Add noise/1
  Angle/1 -> Trigonometric Function/1, Trigonometric Function1/1
  Divide/1 -> New Row/1
  Divide1/1 -> New Row/2
  Trigonometric Function/1 -> Divide3/2, Divide/1
  Trigonometric Function1/1 -> Divide2/1, Divide1/1
  row/1 -> Divide2/2, Divide/2
  col/1 -> Divide1/2, Divide3/1
  Add noise/1 -> Sum of Elements/1
  Center/1 -> Vector Concatenate/1, Vector Concatenate/2, Vector Concatenate/4, Vector Concatenate/3
  Vector Concatenate/1 -> Sum of Elements/2

== system vipmosaicking/Corner Matching/Calculate Distances/For Iterator Subsystem/For Iterator Subsystem/Distance between two feature vectors ==
  f1 : Inport
  f2 : Inport  Port=2
  Abs : Abs
  Add : Sum  Inputs=+-
  Sum of Elements : Sum  Inputs=+
  dis : Outport
  wires:
  Sum of Elements/1 -> dis/1
  Abs/1 -> Sum of Elements/1
  Add/1 -> Abs/1
  f2/1 -> Add/2
  f1/1 -> Add/1

== system vipmosaicking/Corner Matching/Calculate Features/Clip Point Coordinates/Clip row//col coordinates/Clip a Coordinate ==
  Low : Inport
  High : Inport  Port=2
  Coordinate : Inport  Port=3
  MinMax1 : MinMax  Function=max  Inputs=2
  MinMax2 : MinMax  Inputs=2
  Coordinate_clip : Outport
  wires:
  MinMax2/1 -> Coordinate_clip/1
  High/1 -> MinMax2/2
  MinMax1/1 -> MinMax2/1
  Low/1 -> MinMax1/2
  Coordinate/1 -> MinMax1/1

== system vipmosaicking/Input/Synthetic Video Generation/Synthesize Video/Center Locations/Saturate center coordinates ==
  Center : Inport
  Size : Inport  Port=2
  Center2 : Sum  Inputs=-+
  Min Dis to Boundary : Constant  Value=kron([ceil(sqrt(dimen(1)^2+dimen(2)^2)/2)], [1; 1])
  MinMax : MinMax  Function=max  Inputs=2
  MinMax1 : MinMax  Inputs=2
  row1 : Selector  IndexMode=Zero-based  InputPortWidth=3  IndexOptions=Index vector (dialog)  Indices=[0 1]  OutputSizes=1
  Ctr : Outport
  wires:
  Size/1 -> row1/1
  MinMax1/1 -> Ctr/1
  Center/1 -> MinMax/1
  Center2/1 -> MinMax1/2
  MinMax/1 -> MinMax1/1
  row1/1 -> Center2/2
  Min Dis to Boundary/1 -> Center2/1, MinMax/2

== matlab function vipmosaicking/Corner Matching/Calculate Features/Coordinates of the top-left corner of the feature window1 ==
  data: A input; y output size=size(A); V input
function y = fcn(A,V)
%#codegen

s = size(A);
tV = repmat(V',s(1),1);
y = A-tV;
